simulink model "TVC_6DOF_Model_2024a"  (R2024a)
settings: Solver=FixedStepAuto  StartTime=0.0  StopTime=5  FixedStep=.0005  RelTol=1e-3
values from neighbouring files (symbols this model uses):
  init = [0, 0.5, 0]    [quaternionLQR.m]
  K = lqr(A, B, Q, R)    [quaternionLQR.m]
undefined symbols (not defined in the file or in its folder): DiscIntNeverNeededParam, prop
libraries: simulink x4, simulink_extras x1, slpidlib x1, sharedtransform x1, shared6dof x1
settings Model: Creator=lucan  LastModifiedBy=C27Nathan.Aldridge

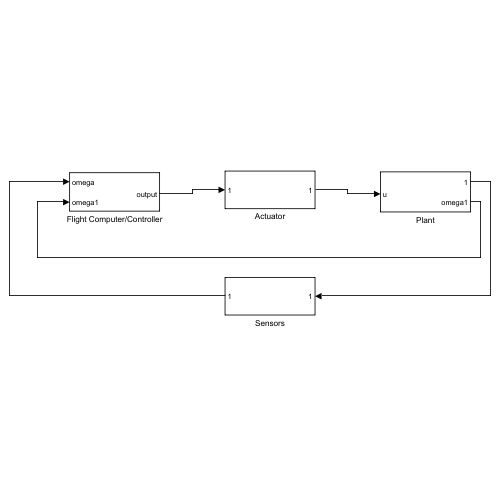
[thumbnail: Simulink's stored preview of the top-level diagram]
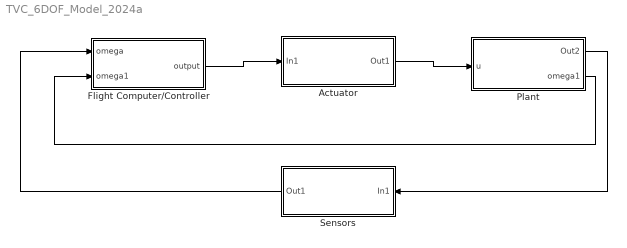
== system TVC_6DOF_Model_2024a ==
  Actuator : Subsystem
  Flight Computer/Controller : Subsystem
  Plant : Subsystem
  Sensors : Subsystem
  wires:
  Plant/1(Out2) -> Sensors/1(In1)
  Sensors/1(Out1) -> Flight Computer/Controller/1(omega)
  Flight Computer/Controller/1(output) -> Actuator/1(In1)
  Actuator/1(Out1) -> Plant/1(u)
  Plant/2(omega1) -> Flight Computer/Controller/2(omega1)

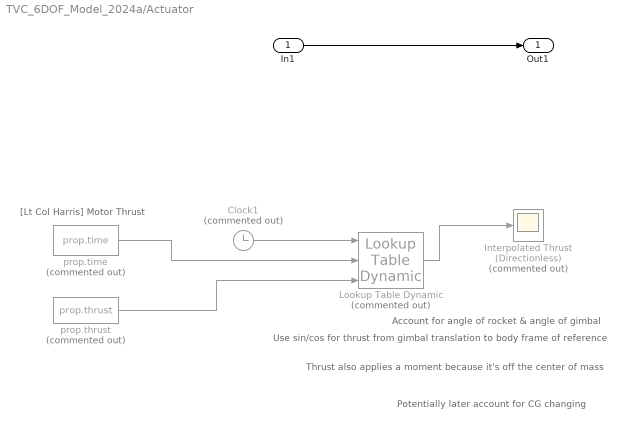
== system TVC_6DOF_Model_2024a/Actuator ==
  note: Potentially later account for CG changing
  note: Thrust also applies a moment because it's off the center of mass
  note: Account for angle of rocket & angle of gimbal
  note: [Lt Col Harris] Motor Thrust
  note: Use sin/cos for thrust from gimbal translation to body frame of reference
  In1 : Inport
  Clock1 : Clock  Commented=on
  Interpolated Thrust (Directionless) : Scope  Commented=on
  Lookup Table Dynamic : simulink/Lookup Tables/Lookup Table Dynamic  Commented=on  LookUpMeth=Interpolation-Use End Values  OutDataType=fixdt('double')  OutScaling=[]  OutputDataTypeScalingMode=Specify via dialog  OutDataTypeStr=double  DoSatur=off
  prop.thrust : Constant  Commented=on  Value=prop.thrust
  prop.time : Constant  Commented=on  Value=prop.time
  Out1 : Outport
  wires:
  In1/1 -> Out1/1
  prop.time/1 -> Lookup Table Dynamic/2
  prop.thrust/1 -> Lookup Table Dynamic/3
  Lookup Table Dynamic/1 -> Interpolated Thrust (Directionless)/1
  Clock1/1 -> Lookup Table Dynamic/1

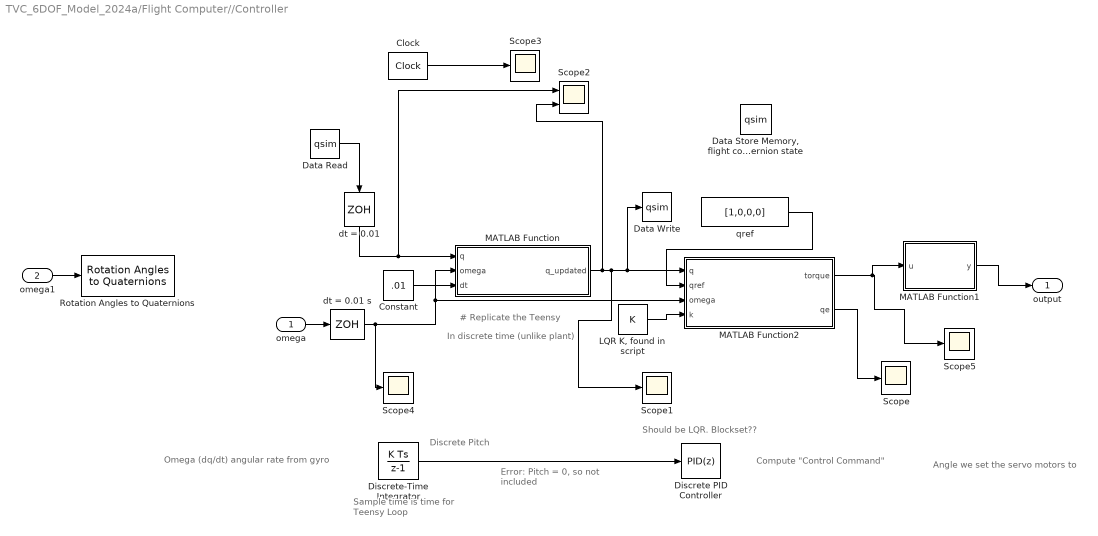
== system TVC_6DOF_Model_2024a/Flight Computer//Controller ==
  note: Angle we set the servo motors to
  note: Error: Pitch = 0, so not included
  note: Should be LQR. Blockset??
  note: Discrete Pitch
  note: Sample time is time for Teensy Loop
  note: In discrete time (unlike plant)
  note: Omega (dq/dt) angular rate from gyro
  note: Compute "Control Command"
  note: # Replicate the Teensy
  omega : Inport
  omega1 : Inport  Port=2
  Clock : simulink_extras/Flip Flops/Clock  period=.01
  Constant : Constant  Value=.01
  Data Read : DataStoreRead  DataStoreName=qsim  IndexOptions=Index vector (dialog)  Indices=1  OutputSizes=1
  "Data Store Memory, flight computer guess of quaternion state" : DataStoreMemory  DataStoreName=qsim  WriteAfterWriteMsg=warning  InitialValue=eul2quat(init, 'XYZ')  ShowAdditionalParam=off
  "Data Write " : DataStoreWrite  DataStoreName=qsim  IndexOptions=Index vector (dialog)  Indices=1  OutputSizes=1
  Discrete PID Controller : slpidlib/PID Controller  Controller=PID  Form=Parallel  TimeDomain=Discrete-time  UseExternalTs=off  SampleTime=-1  IntegratorMethod=Forward Euler  FilterMethod=Forward Euler  ControllerParametersSource=internal  P=1  I=1  UseKiTs=off  D=0  UseExternalDerivativeSource=off  N=100  UseFilter=on  TunerSelectOption=Transfer Function Based (PID Tuner App)  InitialConditionSource=internal  InitialConditionForIntegrator=0  InitialConditionForFilter=0  DifferentiatorICPrevScaledInput=0  ExternalReset=none  TrackingMode=off  Kt=1  LimitOutput=off  SatLimitsSource=internal  UpperSaturationLimit=inf  LowerSaturationLimit=-inf  LinearizeAsGain=off  AntiWindupMode=none  Kb=1  LimitIntegrator=off  UpperIntegratorSaturationLimit=inf  LowerIntegratorSaturationLimit=-inf  POutMin=[]  POutMax=[]  IOutMin=[]  IOutMax=[]  DOutMin=[]  DOutMax=[]  NOutMin=[]  NOutMax=[]  SumOutMin=[]  SumOutMax=[]  SaturationOutMin=[]  SaturationOutMax=[]  PParamMin=[]  PParamMax=[]  IParamMin=[]  IParamMax=[]  DParamMin=[]  DParamMax=[]  NParamMin=[]  NParamMax=[]  KbParamMin=[]  KbParamMax=[]  KtParamMin=[]  KtParamMax=[]  KbOutMin=[]  KbOutMax=[]  KtOutMin=[]  KtOutMax=[]  IntegratorOutMin=[]  IntegratorOutMax=[]  FilterOutMin=[]  FilterOutMax=[]  SumI1OutMin=[]  SumI1OutMax=[]  SumI2OutMin=[]  SumI2OutMax=[]  SumI3OutMin=[]  SumI3OutMax=[]  SumI4OutMin=[]  SumI4OutMax=[]  SumDOutMin=[]  SumDOutMax=[]  DifferentiatorOutMin=[]  DifferentiatorOutMax=[]  FilterDiffOutCoefMin=[]  FilterDiffOutCoefMax=[]  ReciprocalOutMin=[]  ReciprocalOutMax=[]  SumDenOutMin=[]  SumDenOutMax=[]  SumNumOutMin=[]  SumNumOutMax=[]  DivideOutMin=[]  DivideOutMax=[]  UdiffTsProdOutMin=[]  UdiffTsProdOutMax=[]  NTsProdOutMin=[]  NTsProdOutMax=[]  UintegralTsProdOutMin=[]  UintegralTsProdOutMax=[]  UngainTsProdOutMin=[]  UngainTsProdOutMax=[]  ClampingZeroOutDataTypeStr=Inherit: Inherit via back propagation  ClampingZeroOutMin=[]  ClampingZeroOutMax=[]  FilterDenConstantOutDataTypeStr=Inherit: Inherit via back propagation  FilterDenConstantOutMin=[]  FilterDenConstantOutMax=[]  PCopyOutDataTypeStr=Inherit: Inherit via back propagation  PCopyOutMin=[]  PCopyOutMax=[]  NCopyOutDataTypeStr=Inherit: Inherit via back propagation  NCopyOutMin=[]  NCopyOutMax=[]  IntegratorContinuousStateAttributes=''  IntegratorStateMustResolveToSignalObject=off  IntegratorRTWStateStorageClass=Auto  FilterContinuousStateAttributes=''  FilterStateMustResolveToSignalObject=off  FilterRTWStateStorageClass=Auto  ParallelPVariant=InternalParameters  IdealPVariant=Disabled  IVariant=InternalParameters  DVariant=InternalParameters  IntegratorVariant=Discrete  SatVariant=Disabled  AWVariant=Passthrough  PCopyVariant=Disabled  TRVariant=Disabled  FdbkBlocksVariant=Forward  IdealPFdbkVariant=Disabled  SatFdbkVariant=Disabled  DerivativeFilterVariant=ForwardEulerFilter  NVariant=InternalParameters  NCopyVariant=Disabled  FilterICVariant=InternalICsFilter  IntegratorICVariant=InternalICs  ExternalResetVariant=Disabled  TRSumVariant=Passthrough  SumFdbkVariant=Disabled  SumVariant=Sum_PID  TsampFilterVariant=InternalTs  TsampNgainVariant=Passthrough  TsampIntegralVariant=Disabled_SignalSpec  ExternalSaturationOutDataTypeStr=Inherit: Same as second input  DerivativeSourceVariant=ErrorSignal
      settings: LibrarySourceBlock=simulink/Discrete/Discrete PID Controller
  Discrete-Time Integrator : DiscreteIntegrator  SampleTime=0.01  ICPrevOutput=DiscIntNeverNeededParam  ICPrevScaledInput=DiscIntNeverNeededParam
  "LQR K, found in script" : Constant  Value=K
  MATLAB Function : MATLAB Function  TreatAsAtomicUnit=on
  MATLAB Function1 : MATLAB Function  TreatAsAtomicUnit=on
  MATLAB Function2 : MATLAB Function  TreatAsAtomicUnit=on
  Rotation Angles to Quaternions : sharedtransform/Rotation Angles to Quaternions  rotationOrder=XYZ  aMode=aMode
  Scope{,1,3..5} (5 alike) : Scope
  Scope2 : Scope  NumInputPorts=2
  dt = 0.01 : ZeroOrderHold  SampleTime=0.01
  dt = 0.01 s : ZeroOrderHold  SampleTime=0.01
  qref : Constant  Value=[1,0,0,0]
  output : Outport
  wires:
  ? -> Discrete-Time Integrator/1
  Discrete-Time Integrator/1 -> Discrete PID Controller/1
  Constant/1 -> MATLAB Function/3(dt)
  "LQR K, found in script"/1 -> MATLAB Function2/4(k)
  qref/1 -> MATLAB Function2/2(qref)
  omega/1 -> dt = 0.01 s/1
  MATLAB Function2/2(qe) -> Scope/1
  omega1/1 -> Rotation Angles to Quaternions/1
  Clock/1 -> Scope3/1
  Data Read/1 -> dt = 0.01/1
  MATLAB Function/1(q_updated) -> MATLAB Function2/1(q), "Data Write "/1, Scope1/1, Scope2/2
  MATLAB Function2/1(torque) -> MATLAB Function1/1(u), Scope5/1
  dt = 0.01/1 -> MATLAB Function/1(q), Scope2/1
  dt = 0.01 s/1 -> Scope4/1, MATLAB Function2/3(omega), MATLAB Function/2(omega)
  MATLAB Function1/1(y) -> output/1

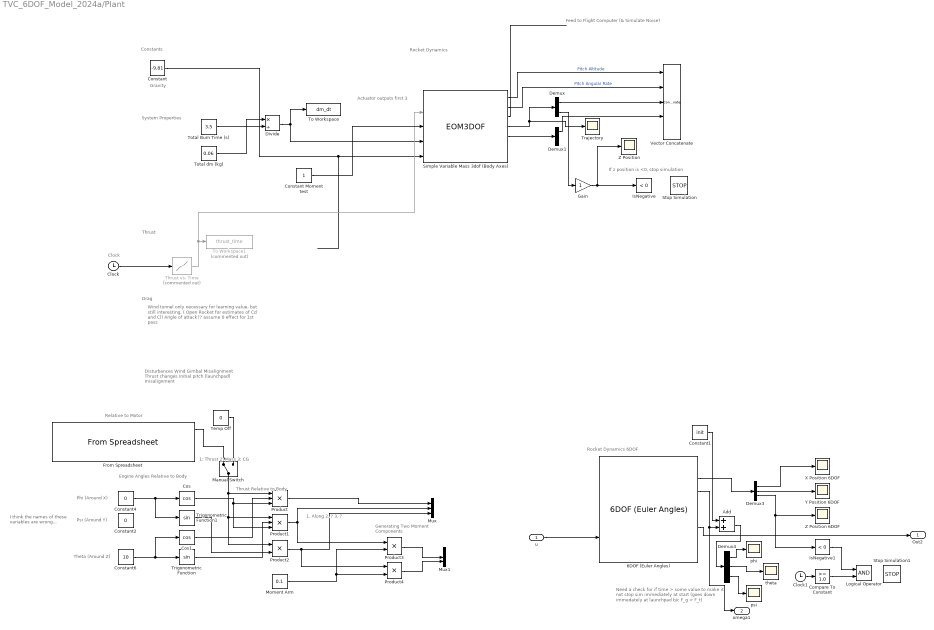
== system TVC_6DOF_Model_2024a/Plant ==
  note: Generating Two
      | Moment Components
  note: I think the names of these
      | variables are wrong...
  note: 1. Along
      | 2. ?
      | 3. ?
  note: Thrust Relative to Body
  note: Phi (Around X)
  note: Psi (Around Y)
  note: Theta (Around Z)
  note: Relative to Motor
  note: Engine Angles Relative to Body
  note: Need a check for if time > some value to make
      | it not stop sim immediately at start (goes down
      | immedately at launchpad b/c F_g > F_t)
  note: 1: Thrust
      | 2: Mass
      | 3: CG
  note: Rocket Dynamics 6DOF
  note: Disturbances
      | Wind
      | Gimbal Misalignment
      | Thrust changes
      | Initial pitch (launchpad) misalignment
  note: Feed to Flight Computer (& Simulate Noise)
  note: Wind tunnel only necessary for learning value, but still interesting. ( Open Rocket for estimates of Cd and Cl)
      |
      | Angle of attack?? assume 0 effect for 1st pass
  note: Actuator outputs first 3
  note: Gravity
  note: Clock
  note: System Properties
  note: If z position is <0, stop simulation
  note: Constants
  note: Rocket Dynamics
  note: Thrust
  note: Drag
  u : Inport
  6DOF (Euler Angles) : shared6dof/6DOF (Euler Angles)  units=Metric (MKS)  mtype=Fixed  rep=Euler Angles  xme_0=[0 0 0]  Vm_0=[0 0 0]  eul_0=[0,0,0]  pm_0=w0  mass_0=1.0  mass_e=0.5  mass_f=2.0  inertia=I  inertia_e=eye(3)  inertia_f=2*eye(3)  k_quat=1.0  vre_flag=on  abi_flag=off  aMode=0  xme_statename=''  Vm_statename=''  eul_statename=''  quat_statename=''  pm_statename=''  mass_statename=''
  Add : Sum
  Clock : Clock
  Clock1 : Clock
  Compare To Constant : simulink/Logic and Bit Operations/Compare To Constant  relop=>=  const=1.0  OutDataTypeStr=boolean
  Constant : Constant  Value=-9.81
  Constant Moment test : Constant
  Constant1 : Constant  Value=init
  Constant2 : Constant  Value=0
  Constant4 : Constant  Value=0
  Constant6 : Constant  Value=10
  Cos : Trigonometry  Operator=cos
  Cos1 : Trigonometry  Operator=cos
  Demux : Demux  Outputs=2
  Demux1 : Demux  Outputs=2
  Demux3 : Demux  Outputs=3
  Demux4 : Demux  Outputs=3
  Divide : Product  Inputs=*/  OutDataTypeStr=double
  From Spreadsheet : FromSpreadsheet  FileName=Mike Haberer F15-0 Thrust Curve.xlsx
  Gain : Gain
  IsNegative : simulink/Logic and Bit Operations/Compare To Zero  relop=<  OutDataTypeStr=boolean
  IsNegative1 : simulink/Logic and Bit Operations/Compare To Zero  relop=<  OutDataTypeStr=boolean
  Logical Operator : Logic  AllPortsSameDT=off  OutDataTypeStr=boolean
  Manual Switch : ManualSwitch
  Moment Arm : Constant  Value=0.1
  Mux : Mux  Inputs=3
  Mux1 : Mux  Inputs=3
  Product : Product  Inputs=3
  Product1 : Product  Inputs=3
  Product2 : Product
  Product3 : Product
  Product4 : Product
  Simple Variable Mass 3dof (Body Axes) : EOM3DOF  mtype=Simple Variable  mass_f=1.0  g_in=External
  Stop Simulation : Stop
  Stop Simulation1 : Stop
  Temp Off : Constant  Value=0
  Thrust vs. Time : Lookup_n-D  Commented=on  NumberOfTableDimensions=1  BreakpointsForDimension1=prop.time  Table=prop.thrust  InternalRulePriority=Speed  RndMeth=Simplest
  To Workspace : ToWorkspace  VariableName=dm_dt  SampleTime=-1
  To Workspace1 : ToWorkspace  Commented=on  VariableName=thrust_time  SampleTime=-1
  Total Burn Time (s) : Constant  Value=3.5
  Total dm (kg) : Constant  Value=0.06
  Trajectory : Scope
  Trigonometric Function : Trigonometry
  Trigonometric Function1 : Trigonometry
  Vector Concatenate : Concatenate  NumInputs=5
  X Position 6DOF : Scope
  Y Position 6DOF : Scope
  Z Position : Scope
  Z Position 6DOF : Scope
  phi : Scope
  psi : Scope
  theta : Scope
  Out2 : Outport
  omega1 : Outport  Port=2
  wires:
  Simple Variable Mass 3dof (Body Axes)/1 -> Vector Concatenate/1  "Pitch Altitude"
  Simple Variable Mass 3dof (Body Axes)/2 -> Vector Concatenate/2  "Pitch Angular Rate"
  Simple Variable Mass 3dof (Body Axes)/5 -> Demux1/1
  Simple Variable Mass 3dof (Body Axes)/4 -> Demux/1, Trajectory/1
  Demux/1 -> Vector Concatenate/3
  Demux1/1 -> Vector Concatenate/4
  Demux/2 -> Gain/1
  Gain/1 -> IsNegative/1, Z Position/1
  Constant/1 -> Simple Variable Mass 3dof (Body Axes)/5
  Divide/1 -> To Workspace/1, Simple Variable Mass 3dof (Body Axes)/4
  Total dm (kg)/1 -> Divide/1
  Total Burn Time (s)/1 -> Divide/2
  Clock/1 -> Thrust vs. Time/1
  Thrust vs. Time/1 -> To Workspace1/1, Simple Variable Mass 3dof (Body Axes)/2
  Constant Moment test/1 -> Simple Variable Mass 3dof (Body Axes)/3
  Simple Variable Mass 3dof (Body Axes)/3 -> ?
  6DOF (Euler Angles)/2 -> Demux3/1
  Demux3/3 -> IsNegative1/1, Z Position 6DOF/1
  Product1/1 -> Product3/1, Mux/2
  Manual Switch/1 -> Product/1, Product2/1, Product1/1
  Product/1 -> Mux/1
  Demux3/1 -> X Position 6DOF/1
  Demux3/2 -> Y Position 6DOF/1
  Constant6/1 -> Cos1/1, Trigonometric Function/1
  Constant4/1 -> Trigonometric Function1/1, Cos/1
  Cos/1 -> Product/3, Product1/3
  Cos1/1 -> Product/2
  Trigonometric Function/1 -> Product1/2
  Trigonometric Function1/1 -> Product2/2
  Product2/1 -> Product4/1, Mux/3
  Clock1/1 -> Compare To Constant/1
  Compare To Constant/1 -> Logical Operator/2
  IsNegative1/1 -> Logical Operator/1
  Temp Off/1 -> Manual Switch/2
  From Spreadsheet/1 -> Manual Switch/1
  Moment Arm/1 -> Product3/2, Product4/2
  Product4/1 -> Mux1/3
  Product3/1 -> Mux1/2
  Demux4/1 -> phi/1
  Demux4/2 -> theta/1
  Demux4/3 -> psi/1
  u/1 -> 6DOF (Euler Angles)/2
  6DOF (Euler Angles)/3 -> Add/2, omega1/1
  Constant1/1 -> Add/1
  Add/1 -> Demux4/1
  6DOF (Euler Angles)/6 -> Out2/1

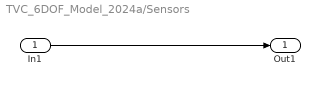
== system TVC_6DOF_Model_2024a/Sensors ==
  In1 : Inport
  Out1 : Outport
  wires:
  In1/1 -> Out1/1

== matlab function TVC_6DOF_Model_2024a/Flight Computer//Controller/MATLAB Function1 ==
  data: u input; y output
function y = fcn(u)
y = [0, u(2), u(3)];
end

== matlab function TVC_6DOF_Model_2024a/Flight Computer//Controller/MATLAB Function ==
  data: q input; q_updated output; omega input; dt input
function q_updated = update_quaternion(q, omega, dt)
    % q: Current quaternion [w, x, y, z]
    q = [q(1), q(2), q(3), q(4)];
    %ensure w is a row vector
    w = [omega(1), omega(2), omega(3)];
    A = [0 -w(1) -w(2) -w(3);
        w(1) 0 w(3) -w(2);
        w(2) -w(3) 0 w(1);
        w(3) w(2) -w(1) 0];
    B = [q(1) -q(2) -q(3) -q(4);
        q(2) q(1) -q(4) q(3);
        q(3) q(4) q(1) -q(2);
        q(4) -q(3) q(2) q(1)];

   qdot = 0.5*A*q';

   q_updated = q+(qdot*dt)';

    % Normalize to prevent drift
    q_updated = q_updated / norm(q_updated);
end

== matlab function TVC_6DOF_Model_2024a/Flight Computer//Controller/MATLAB Function2 ==
  data: q input; torque output; qref input; omega input; k input; qe output
function [torque,qe] = quaternion_control_law(q, qref, omega, k)
    % Compute the conjugate of the quaternion
    q = [q(1), q(2), q(3), q(4)];
    qref_conj = [qref(1), -qref(2), -qref(3), -qref(4)];

    %compute norm
    norm_squared = qref(1)^2 + qref(2)^2 + qref(3)^2 + qref(4)^2;

    % Compute the inverse of the quaternion
    qref_inv = qref_conj / norm_squared;
    
    %find qe
    qe = quatmultiply(qref_inv, q);
    % qe = q;

    %take the last 3 elements of q as used in the state space and the omega
    torque = -k*[[qe(2); qe(3); qe(4)]; omega];
end
